simulink library "variableBuoyancy"  (R2018b)
settings: Solver=VariableStepAuto  StartTime=0.0  StopTime=10.0  RelTol=1e-3
values from neighbouring files (symbols this model uses):
  grav = 9.81    [simpSubPlatform_ts.m]
  h = vol^(1/3)    (= 1.51829448594)    [simpSubPlatform_ts.m]
  oceanDepth = 100+ h/4    (= 100.379573621)    [simpSubPlatform_ts.m]
  rho = 1000    [simpSubPlatform_ts.m]
  vol = 3.5    [simpSubPlatform_ts.m]
  waveAmp = 3    [simpSubPlatform_ts.m]
  wavePeriod = oceanPeriod    (= 20)    [simpSubPlatform_ts.m]
libraries: dspstat3 x1
settings Model: Creator=Erin B  LastModifiedBy=Erin B

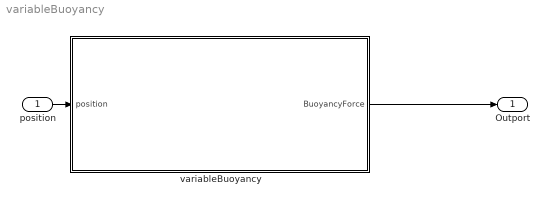
== system variableBuoyancy ==
  position : Inport
  variableBuoyancy : Subsystem  mask{vol=vol, h=h, grav=grav, rho=rho, waveAmplitude=waveAmp, oceanDepth=oceanDepth, wavePeriod=wavePeriod}
      mask prompts: vol "Volume"; h "Height of Object"; grav "Gravity"; rho "Density of Fluid"; waveAmplitude "Wave Amplitude"; oceanDepth "Ocean Depth"; wavePeriod "Wave Period"
  Outport : Outport
  wires:
  variableBuoyancy/1(BuoyancyForce) -> Outport/1
  position/1 -> variableBuoyancy/1(position)

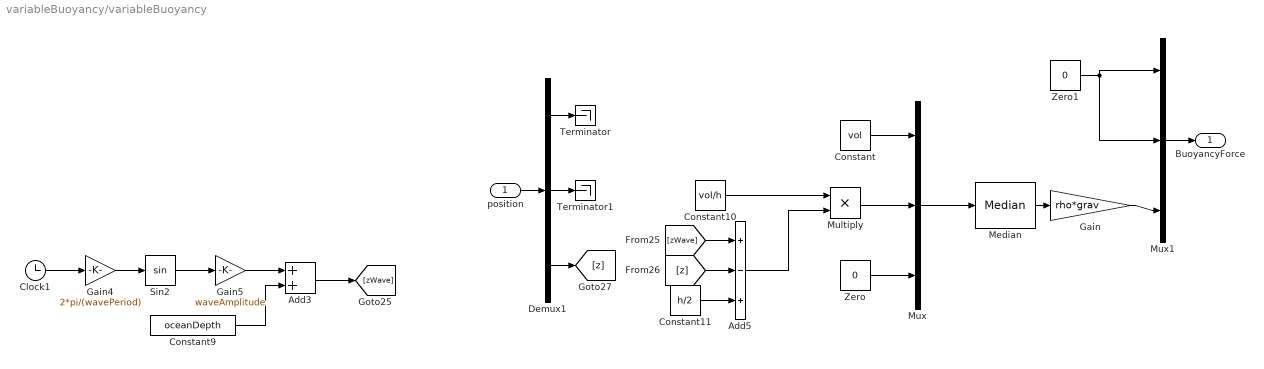
== system variableBuoyancy/variableBuoyancy ==
  position : Inport
  Add3 : Sum
  Add5 : Sum  Inputs=+-+
  Clock1 : Clock
  Constant : Constant  Value=vol
  Constant10 : Constant  Value=vol/h
  Constant11 : Constant  Value=h/2
  Constant9 : Constant  Value=oceanDepth
  Demux1 : Demux  Outputs=3
  Gain : Gain  Gain=rho*grav
  Gain4 : Gain  Gain=2*pi/(wavePeriod)
  Gain5 : Gain  Gain=waveAmplitude
  Median : dspstat3/Median  sortAlg=Quick sort  directionMode=Each column  dimension=1  roundingMode=Floor  overflowMode=off  accumDataTypeStr=Inherit: Same as product output  accumLastDataTypeStr=Inherit: Same as product output  outputDataTypeStr=Inherit: Same as accumulator  outputMin=[]  outputMax=[]  outputLastDataTypeStr=Inherit: Same as accumulator
      settings: SourceProductName=DSP System Toolbox  SourceProductBaseCode=DS  allowOverrides=off
  Multiply : Product
  Mux : Mux  Inputs=3
  Mux1 : Mux  Inputs=3
  Sin2 : Trigonometry
  Terminator : Terminator
  Terminator1 : Terminator
  Zero : Constant  Value=0  OutDataTypeStr=Inherit: Inherit via back propagation
  Zero1 : Constant  Value=0  OutDataTypeStr=Inherit: Inherit via back propagation
  BuoyancyForce : Outport
  wires:
  Gain4/1 -> Sin2/1
  Median/1 -> Gain/1
  Add5/1 -> Multiply/2
  [zWave] -> Add5/1
  Constant9/1 -> Add3/2
  Constant11/1 -> Add5/3
  [z] -> Add5/2
  Gain5/1 -> Add3/1
  Clock1/1 -> Gain4/1
  Demux1/3 -> [z]
  Constant10/1 -> Multiply/1
  Add3/1 -> [zWave]
  Sin2/1 -> Gain5/1
  Mux/1 -> Median/1
  Constant/1 -> Mux/1
  Multiply/1 -> Mux/2
  Zero/1 -> Mux/3
  Demux1/1 -> Terminator/1
  Demux1/2 -> Terminator1/1
  position/1 -> Demux1/1
  Gain/1 -> Mux1/3
  Mux1/1 -> BuoyancyForce/1
  Zero1/1 -> Mux1/2, Mux1/1
